simulink model "bh_4dof_LAGR_manipulator"  (R2016a)
settings: Solver=ode15s  StartTime=0.0  StopTime=30  FixedStep=0.001  RelTol=1e-5
values from neighbouring files (symbols this model uses):
  b1_damp = 0.005    [bh_params_single_link_control_explore.m]
  b4_damp = 0.005    [bh_params_single_link_control_explore.m]
  g = 9.80665    [bh_params_single_link_control_explore.m]
  Hz = 0.20    (= 0.2)    [bh_params_single_link_control_explore.m]
  L1x = 1.5    [bh_params_single_link_control_explore.m]
  L1y = 0.050    (= 0.05)    [bh_params_single_link_control_explore.m]
  L1z = 0.005    [bh_params_single_link_control_explore.m]
  mass1 = density * L1x*L1y*L1z    (= 0.375)    [bh_params_single_link_control_explore.m]
  mass4 = density * Hz*pi*(Rturn^2)    (= 1.57079632679)    [bh_params_single_link_control_explore.m]
  Rturn = 0.05    [bh_params_single_link_control_explore.m]
  theta1_0 = 0    [bh_params_single_link_control_explore.m]
  theta1_dot_0 = 0    [bh_params_single_link_control_explore.m]
  theta4_0 = 0    [bh_params_single_link_control_explore.m]
  theta4_dot_0 = 0    [bh_params_single_link_control_explore.m]
undefined symbols (not defined in the file or in its folder): b2_damp, b3_damp, L2x, L2y, L2z, L3x, L3y, L3z, mass2, mass3, theta2_0, theta2_dot_0, theta3_0, theta3_dot_0, X, Y, Z
libraries: sm_lib x26, nesl_utility x17
(part 1 of 2)
settings Model: Creator=bhorton  LastModifiedBy=bhorton
settings SolverCC: ZeroCrossAlgorithm=Adaptive
settings GRTTargetCC: GeneratePreprocessorConditionals=Use local settings
settings SimscapeCC: SimscapeLogType=all  SimscapeLogDataHistory=10000  SelectedTab=Simscape Multibody

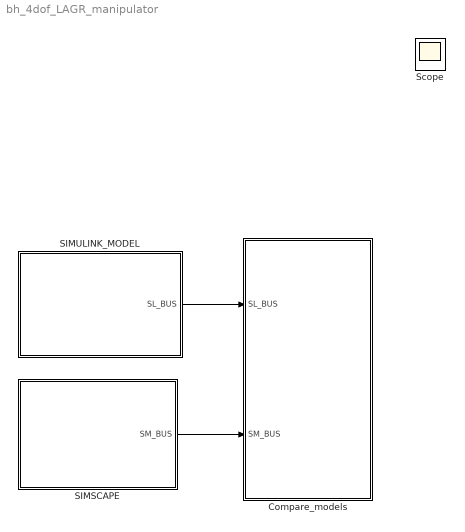
== system bh_4dof_LAGR_manipulator ==
  Compare_models : Subsystem
  SIMSCAPE : Subsystem
  SIMULINK_MODEL : Subsystem
  Scope : Scope
  wires:
  SIMULINK_MODEL/1(SL_BUS) -> Compare_models/1(SL_BUS)
  SIMSCAPE/1(SM_BUS) -> Compare_models/2(SM_BUS)

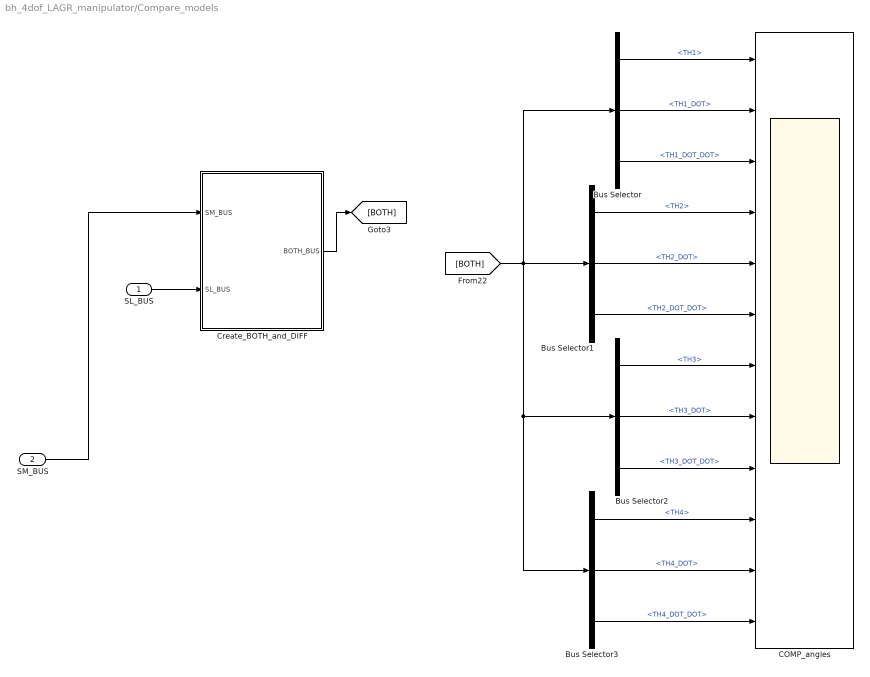
== system bh_4dof_LAGR_manipulator/Compare_models ==
  SL_BUS : Inport
  SM_BUS : Inport  Port=2
  Bus Selector : BusSelector  OutputSignals=TH1,TH1_DOT,TH1_DOT_DOT
  Bus Selector1 : BusSelector  OutputSignals=TH2,TH2_DOT,TH2_DOT_DOT
  Bus Selector2 : BusSelector  OutputSignals=TH3,TH3_DOT,TH3_DOT_DOT
  Bus Selector3 : BusSelector  OutputSignals=TH4,TH4_DOT,TH4_DOT_DOT
  COMP_angles : Scope  NumInputPorts=12
  Create_BOTH_and_DIFF : Subsystem
  wires:
  SM_BUS/1 -> Create_BOTH_and_DIFF/1(SM_BUS)
  SL_BUS/1 -> Create_BOTH_and_DIFF/2(SL_BUS)
  Create_BOTH_and_DIFF/1(BOTH_BUS) -> [BOTH]
  Bus Selector/1 -> COMP_angles/1  "<TH1>"
  Bus Selector/2 -> COMP_angles/2  "<TH1_DOT>"
  Bus Selector/3 -> COMP_angles/3  "<TH1_DOT_DOT>"
  Bus Selector1/1 -> COMP_angles/4  "<TH2>"
  Bus Selector1/2 -> COMP_angles/5  "<TH2_DOT>"
  Bus Selector1/3 -> COMP_angles/6  "<TH2_DOT_DOT>"
  Bus Selector2/1 -> COMP_angles/7  "<TH3>"
  Bus Selector2/2 -> COMP_angles/8  "<TH3_DOT>"
  Bus Selector2/3 -> COMP_angles/9  "<TH3_DOT_DOT>"
  [BOTH] -> Bus Selector/1, Bus Selector3/1, Bus Selector2/1, Bus Selector1/1
  Bus Selector3/1 -> COMP_angles/10  "<TH4>"
  Bus Selector3/2 -> COMP_angles/11  "<TH4_DOT>"
  Bus Selector3/3 -> COMP_angles/12  "<TH4_DOT_DOT>"

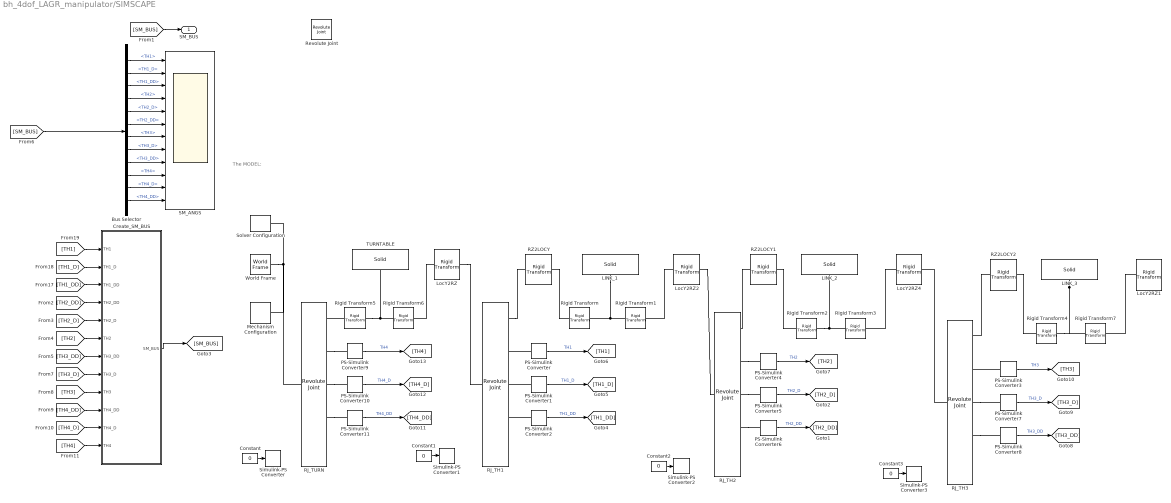
== system bh_4dof_LAGR_manipulator/SIMSCAPE ==
  note: The MODEL:
  Bus Selector : BusSelector  OutputSignals=TH1,TH1_D,TH1_DD,TH2,TH2_D,TH2_DD,TH3,TH3_D,TH3_DD,TH4,TH4_D,TH4_DD
  Constant{,1..3} (4 alike) : Constant  Value=0
  Create_SM_BUS : Subsystem
  LINK_1 : sm_lib/Body Elements/Solid  InertiaType=CalculateFromGeometry  Mass=1  MassUnits=kg  CenterOfMass=[0 0 0]  CenterOfMassUnits=m  MomentsOfInertia=[1 1 1]  MomentsOfInertiaUnits=kg*m^2  ProductsOfInertia=[0 0 0]  ProductsOfInertiaUnits=kg*m^2  DensityBased=on  Density=density  DensityUnits=kg/(m^3)  DoExposeReferenceFrame=on  SerializedFrames=<Frames/>  GraphicType=FromGeometry  MarkerShape=Sphere  MarkerSize=10  GraphicVisPropType=SimpleVisualProperties  GraphicDiffuseColor=[0.2 0.2 1.0]  GraphicSpecularColor=[0.5 0.5 0.5 1.0]  GraphicAmbientColor=[0.15 0.15 0.15 1.0]  GraphicEmissiveColor=[0.0 0.0 0.0 1.0]  GraphicShininess=75  GraphicOpacity=1.0  GeometryShape=Brick  RectangleSize=[1 1]  RectangleSizeUnits=m  BrickDimensions=[L1x, L1y, L1z ]  BrickDimensionUnits=m  CylinderRadius=1  CylinderRadiusUnits=m  CylinderLength=1  CylinderLengthUnits=m  SphereRadius=1  SphereRadiusUnits=m  EllipsoidRadii=[1 1 1]  EllipsoidRadiiUnits=m  ExtrusionCrossSection=[1 1; -1 1; -1 -1; 1 -1]  ExtrusionCrossSectionUnits=m  ExtrusionLength=1  ExtrusionLengthUnits=m  PolygonNumSides=3  PolygonOuterRadius=1  PolygonOuterRadiusUnits=m  ExtGeomFileType=STEP  ExtGeomFileUnits=m  RevolutionCrossSection=[1 1; 1 -1; 2 -1; 2 1]  RevolutionCrossSectionUnits=m  RevolutionExtent=Full  RevolutionAngle=180  RevolutionAngleUnits=deg
  LINK_2 : sm_lib/Body Elements/Solid  InertiaType=CalculateFromGeometry  Mass=1  MassUnits=kg  CenterOfMass=[0 0 0]  CenterOfMassUnits=m  MomentsOfInertia=[1 1 1]  MomentsOfInertiaUnits=kg*m^2  ProductsOfInertia=[0 0 0]  ProductsOfInertiaUnits=kg*m^2  DensityBased=on  Density=density  DensityUnits=kg/(m^3)  DoExposeReferenceFrame=on  SerializedFrames=<Frames/>  GraphicType=FromGeometry  MarkerShape=Sphere  MarkerSize=10  GraphicVisPropType=SimpleVisualProperties  GraphicDiffuseColor=[0.8 0.8 1.0]  GraphicSpecularColor=[0.5 0.5 0.5 1.0]  GraphicAmbientColor=[0.15 0.15 0.15 1.0]  GraphicEmissiveColor=[0.0 0.0 0.0 1.0]  GraphicShininess=75  GraphicOpacity=1.0  GeometryShape=Brick  RectangleSize=[1 1]  RectangleSizeUnits=m  BrickDimensions=[L2x, L2y, L2z ]  BrickDimensionUnits=m  CylinderRadius=1  CylinderRadiusUnits=m  CylinderLength=1  CylinderLengthUnits=m  SphereRadius=1  SphereRadiusUnits=m  EllipsoidRadii=[1 1 1]  EllipsoidRadiiUnits=m  ExtrusionCrossSection=[1 1; -1 1; -1 -1; 1 -1]  ExtrusionCrossSectionUnits=m  ExtrusionLength=1  ExtrusionLengthUnits=m  PolygonNumSides=3  PolygonOuterRadius=1  PolygonOuterRadiusUnits=m  ExtGeomFileType=STEP  ExtGeomFileUnits=m  RevolutionCrossSection=[1 1; 1 -1; 2 -1; 2 1]  RevolutionCrossSectionUnits=m  RevolutionExtent=Full  RevolutionAngle=180  RevolutionAngleUnits=deg
  LINK_3 : sm_lib/Body Elements/Solid  InertiaType=CalculateFromGeometry  Mass=1  MassUnits=kg  CenterOfMass=[0 0 0]  CenterOfMassUnits=m  MomentsOfInertia=[1 1 1]  MomentsOfInertiaUnits=kg*m^2  ProductsOfInertia=[0 0 0]  ProductsOfInertiaUnits=kg*m^2  DensityBased=on  Density=density  DensityUnits=kg/(m^3)  DoExposeReferenceFrame=on  SerializedFrames=<Frames/>  GraphicType=FromGeometry  MarkerShape=Sphere  MarkerSize=10  GraphicVisPropType=SimpleVisualProperties  GraphicDiffuseColor=[1.0 0.8 0.4]  GraphicSpecularColor=[0.5 0.5 0.5 1.0]  GraphicAmbientColor=[0.15 0.15 0.15 1.0]  GraphicEmissiveColor=[0.0 0.0 0.0 1.0]  GraphicShininess=75  GraphicOpacity=1.0  GeometryShape=Brick  RectangleSize=[1 1]  RectangleSizeUnits=m  BrickDimensions=[L3x, L3y, L3z ]  BrickDimensionUnits=m  CylinderRadius=1  CylinderRadiusUnits=m  CylinderLength=1  CylinderLengthUnits=m  SphereRadius=1  SphereRadiusUnits=m  EllipsoidRadii=[1 1 1]  EllipsoidRadiiUnits=m  ExtrusionCrossSection=[1 1; -1 1; -1 -1; 1 -1]  ExtrusionCrossSectionUnits=m  ExtrusionLength=1  ExtrusionLengthUnits=m  PolygonNumSides=3  PolygonOuterRadius=1  PolygonOuterRadiusUnits=m  ExtGeomFileType=STEP  ExtGeomFileUnits=m  RevolutionCrossSection=[1 1; 1 -1; 2 -1; 2 1]  RevolutionCrossSectionUnits=m  RevolutionExtent=Full  RevolutionAngle=180  RevolutionAngleUnits=deg
  LocY2RZ{,1..2,4} (4 alike) : sm_lib/Frames and Transforms/Rigid Transform  TranslationMethod=None  TranslationLengthUnit=m  TranslationStandardAxis=+Z  TranslationStandardOffset=Hz/2  TranslationCartesianOffset=[0 0 0]  TranslationROffset=0  TranslationROffsetUnits=m  TranslationZOffset=0  TranslationZOffsetUnits=m  TranslationThetaOffset=0  TranslationThetaOffsetUnits=deg  RotationMethod=AlignedAxes  RotationAngleUnits=deg  RotationStandardAxis=+Z  RotationAngle=0.0  RotationArbitraryAxis=[0 0 1]  FollAlignAxisA=+X  BaseAlignAxisA=+Y  FollAlignAxisB=+Y  BaseAlignAxisB=+Z  RotationSequenceAxes=FollowerAxes  RotationSequence=XYX  RotationSequenceAngles=[0 0 0]  RotationSequenceAnglesUnits=deg  RotationMatrix=[1 0 0; 0 1 0; 0 0 1]
  Mechanism Configuration : sm_lib/Utilities/Mechanism Configuration  UniformGravity=Constant  GravityVector=[0 0 -9.80665 ]  GravityUnits=m/s^2  LinearizationDelta=1e-4
  PS-Simulink Converter{,3..4,9} (4 alike) : nesl_utility/PS-Simulink Converter  PhysicalDomain=network_engine_domain  SubClassName=ps_output  LeftPortType=input  RightPortType=output  PseudoPeriodic=off  Frequencies=[]  Unit=rad  AffineConversion=off
  PS-Simulink Converter{1,5,7,10} (4 alike) : nesl_utility/PS-Simulink Converter  PhysicalDomain=network_engine_domain  SubClassName=ps_output  LeftPortType=input  RightPortType=output  PseudoPeriodic=off  Frequencies=[]  Unit=rad/s  AffineConversion=off
  PS-Simulink Converter{2,6,8,11} (4 alike) : nesl_utility/PS-Simulink Converter  PhysicalDomain=network_engine_domain  SubClassName=ps_output  LeftPortType=input  RightPortType=output  PseudoPeriodic=off  Frequencies=[]  Unit=rad/s^2  AffineConversion=off
  RJ_TH1 : sm_lib/Joints/Revolute Joint  SenseConstraintForce=on  SenseConstraintForceX=off  SenseConstraintForceY=off  SenseConstraintForceZ=off  SenseConstraintTorque=off  SenseConstraintTorqueX=off  SenseConstraintTorqueY=off  SenseConstraintTorqueZ=off  SenseTotalForce=off  SenseTotalForceX=off  SenseTotalForceY=off  SenseTotalForceZ=off  SenseTotalTorque=off  SenseTotalTorqueX=off  SenseTotalTorqueY=off  SenseTotalTorqueZ=off  CompositeWrenchDir=BaseOnFollower  CompositeWrenchFrame=BaseFrame  EquilibriumPosition=0  EquilibriumPositionUnits=deg  SpringStiffness=0  SpringStiffnessUnits=N*m/deg  DampingCoefficient=b1_damp  DampingCoefficientUnits=N*m/(rad/s)  TorqueActuationMode=NoTorque  MotionActuationMode=ComputedMotion  SensePosition=on  SenseVelocity=on  SenseAcceleration=on  SenseTorqueForce=off  PositionTargetSpecify=on  PositionTargetPriority=Low  PositionTargetValue=theta1_0  PositionTargetValueUnits=rad  VelocityTargetSpecify=on  VelocityTargetPriority=High  VelocityTargetValue=theta1_dot_0  VelocityTargetValueUnits=rad/s
      settings: AttributesFormatString=|
      | %<DampingCoefficient>
      | %<PositionTargetValue>
      | %<VelocityTargetValue>
  RJ_TH2 : sm_lib/Joints/Revolute Joint  SenseConstraintForce=on  SenseConstraintForceX=off  SenseConstraintForceY=off  SenseConstraintForceZ=off  SenseConstraintTorque=off  SenseConstraintTorqueX=off  SenseConstraintTorqueY=off  SenseConstraintTorqueZ=off  SenseTotalForce=off  SenseTotalForceX=off  SenseTotalForceY=off  SenseTotalForceZ=off  SenseTotalTorque=off  SenseTotalTorqueX=off  SenseTotalTorqueY=off  SenseTotalTorqueZ=off  CompositeWrenchDir=BaseOnFollower  CompositeWrenchFrame=BaseFrame  EquilibriumPosition=0  EquilibriumPositionUnits=deg  SpringStiffness=0  SpringStiffnessUnits=N*m/deg  DampingCoefficient=b2_damp  DampingCoefficientUnits=N*m/(rad/s)  TorqueActuationMode=NoTorque  MotionActuationMode=ComputedMotion  SensePosition=on  SenseVelocity=on  SenseAcceleration=on  SenseTorqueForce=off  PositionTargetSpecify=on  PositionTargetPriority=Low  PositionTargetValue=theta2_0  PositionTargetValueUnits=rad  VelocityTargetSpecify=on  VelocityTargetPriority=High  VelocityTargetValue=theta2_dot_0  VelocityTargetValueUnits=rad/s
      settings: AttributesFormatString=|
      | %<DampingCoefficient>
      | %<PositionTargetValue>
      | %<VelocityTargetValue>
  RJ_TH3 : sm_lib/Joints/Revolute Joint  SenseConstraintForce=on  SenseConstraintForceX=off  SenseConstraintForceY=off  SenseConstraintForceZ=off  SenseConstraintTorque=off  SenseConstraintTorqueX=off  SenseConstraintTorqueY=off  SenseConstraintTorqueZ=off  SenseTotalForce=off  SenseTotalForceX=off  SenseTotalForceY=off  SenseTotalForceZ=off  SenseTotalTorque=off  SenseTotalTorqueX=off  SenseTotalTorqueY=off  SenseTotalTorqueZ=off  CompositeWrenchDir=BaseOnFollower  CompositeWrenchFrame=BaseFrame  EquilibriumPosition=0  EquilibriumPositionUnits=deg  SpringStiffness=0  SpringStiffnessUnits=N*m/deg  DampingCoefficient=b3_damp  DampingCoefficientUnits=N*m/(rad/s)  TorqueActuationMode=NoTorque  MotionActuationMode=ComputedMotion  SensePosition=on  SenseVelocity=on  SenseAcceleration=on  SenseTorqueForce=off  PositionTargetSpecify=on  PositionTargetPriority=Low  PositionTargetValue=theta3_0  PositionTargetValueUnits=rad  VelocityTargetSpecify=on  VelocityTargetPriority=High  VelocityTargetValue=theta3_dot_0  VelocityTargetValueUnits=rad/s
      settings: AttributesFormatString=|
      | %<DampingCoefficient>
      | %<PositionTargetValue>
      | %<VelocityTargetValue>
  RJ_TURN : sm_lib/Joints/Revolute Joint  SenseConstraintForce=on  SenseConstraintForceX=off  SenseConstraintForceY=off  SenseConstraintForceZ=off  SenseConstraintTorque=off  SenseConstraintTorqueX=off  SenseConstraintTorqueY=off  SenseConstraintTorqueZ=off  SenseTotalForce=off  SenseTotalForceX=off  SenseTotalForceY=off  SenseTotalForceZ=off  SenseTotalTorque=off  SenseTotalTorqueX=off  SenseTotalTorqueY=off  SenseTotalTorqueZ=off  CompositeWrenchDir=BaseOnFollower  CompositeWrenchFrame=BaseFrame  EquilibriumPosition=0  EquilibriumPositionUnits=deg  SpringStiffness=0  SpringStiffnessUnits=N*m/deg  DampingCoefficient=b4_damp  DampingCoefficientUnits=N*m/(rad/s)  TorqueActuationMode=NoTorque  MotionActuationMode=ComputedMotion  SensePosition=on  SenseVelocity=on  SenseAcceleration=on  SenseTorqueForce=off  PositionTargetSpecify=on  PositionTargetPriority=Low  PositionTargetValue=theta4_0  PositionTargetValueUnits=rad  VelocityTargetSpecify=on  VelocityTargetPriority=High  VelocityTargetValue=theta4_dot_0  VelocityTargetValueUnits=rad/s
      settings: AttributesFormatString=|
      | %<DampingCoefficient>
      | %<PositionTargetValue>
      | %<VelocityTargetValue>
  RZ2LOCY : sm_lib/Frames and Transforms/Rigid Transform  TranslationMethod=None  TranslationLengthUnit=m  TranslationStandardAxis=+Z  TranslationStandardOffset=Hz/2  TranslationCartesianOffset=[0 0 0]  TranslationROffset=0  TranslationROffsetUnits=m  TranslationZOffset=0  TranslationZOffsetUnits=m  TranslationThetaOffset=0  TranslationThetaOffsetUnits=deg  RotationMethod=AlignedAxes  RotationAngleUnits=deg  RotationStandardAxis=+Z  RotationAngle=0.0  RotationArbitraryAxis=[0 0 1]  FollAlignAxisA=+Y  BaseAlignAxisA=+X  FollAlignAxisB=+X  BaseAlignAxisB=+Z  RotationSequenceAxes=FollowerAxes  RotationSequence=XYX  RotationSequenceAngles=[0 0 0]  RotationSequenceAnglesUnits=deg  RotationMatrix=[1 0 0; 0 1 0; 0 0 1]
  RZ2LOCY1 : sm_lib/Frames and Transforms/Rigid Transform  TranslationMethod=None  TranslationLengthUnit=m  TranslationStandardAxis=+Z  TranslationStandardOffset=Hz/2  TranslationCartesianOffset=[0 0 0]  TranslationROffset=0  TranslationROffsetUnits=m  TranslationZOffset=0  TranslationZOffsetUnits=m  TranslationThetaOffset=0  TranslationThetaOffsetUnits=deg  RotationMethod=AlignedAxes  RotationAngleUnits=deg  RotationStandardAxis=+Z  RotationAngle=0.0  RotationArbitraryAxis=[0 0 1]  FollAlignAxisA=+Y  BaseAlignAxisA=+X  FollAlignAxisB=+X  BaseAlignAxisB=+Z  RotationSequenceAxes=FollowerAxes  RotationSequence=XYX  RotationSequenceAngles=[0 0 0]  RotationSequenceAnglesUnits=deg  RotationMatrix=[1 0 0; 0 1 0; 0 0 1]
  RZ2LOCY2 : sm_lib/Frames and Transforms/Rigid Transform  TranslationMethod=None  TranslationLengthUnit=m  TranslationStandardAxis=+Z  TranslationStandardOffset=Hz/2  TranslationCartesianOffset=[0 0 0]  TranslationROffset=0  TranslationROffsetUnits=m  TranslationZOffset=0  TranslationZOffsetUnits=m  TranslationThetaOffset=0  TranslationThetaOffsetUnits=deg  RotationMethod=AlignedAxes  RotationAngleUnits=deg  RotationStandardAxis=+Z  RotationAngle=0.0  RotationArbitraryAxis=[0 0 1]  FollAlignAxisA=+Y  BaseAlignAxisA=+X  FollAlignAxisB=+X  BaseAlignAxisB=+Z  RotationSequenceAxes=FollowerAxes  RotationSequence=XYX  RotationSequenceAngles=[0 0 0]  RotationSequenceAnglesUnits=deg  RotationMatrix=[1 0 0; 0 1 0; 0 0 1]
  Revolute Joint : sm_lib/Joints/Revolute Joint  SenseConstraintForce=off  SenseConstraintForceX=off  SenseConstraintForceY=off  SenseConstraintForceZ=off  SenseConstraintTorque=off  SenseConstraintTorqueX=off  SenseConstraintTorqueY=off  SenseConstraintTorqueZ=off  SenseTotalForce=off  SenseTotalForceX=off  SenseTotalForceY=off  SenseTotalForceZ=off  SenseTotalTorque=off  SenseTotalTorqueX=off  SenseTotalTorqueY=off  SenseTotalTorqueZ=off  CompositeWrenchDir=FollowerOnBase  CompositeWrenchFrame=BaseFrame  EquilibriumPosition=0  EquilibriumPositionUnits=deg  SpringStiffness=0  SpringStiffnessUnits=N*m/deg  DampingCoefficient=0  DampingCoefficientUnits=N*m/(deg/s)  TorqueActuationMode=NoTorque  MotionActuationMode=ComputedMotion  SensePosition=off  SenseVelocity=off  SenseAcceleration=off  SenseTorqueForce=off  PositionTargetSpecify=off  PositionTargetPriority=High  PositionTargetValue=0  PositionTargetValueUnits=deg  VelocityTargetSpecify=off  VelocityTargetPriority=High  VelocityTargetValue=0  VelocityTargetValueUnits=deg/s
  Rigid Transform : sm_lib/Frames and Transforms/Rigid Transform  TranslationMethod=StandardAxis  TranslationLengthUnit=m  TranslationStandardAxis=+Y  TranslationStandardOffset=L1y/2  TranslationCartesianOffset=[0 0 0]  TranslationROffset=0  TranslationROffsetUnits=m  TranslationZOffset=0  TranslationZOffsetUnits=m  TranslationThetaOffset=0  TranslationThetaOffsetUnits=deg  RotationMethod=None  RotationAngleUnits=deg  RotationStandardAxis=+Z  RotationAngle=0.0  RotationArbitraryAxis=[0 0 1]  FollAlignAxisA=+X  BaseAlignAxisA=+Y  FollAlignAxisB=+Y  BaseAlignAxisB=+Z  RotationSequenceAxes=FollowerAxes  RotationSequence=XYX  RotationSequenceAngles=[0 0 0]  RotationSequenceAnglesUnits=deg  RotationMatrix=[1 0 0; 0 1 0; 0 0 1]
  Rigid Transform1 : sm_lib/Frames and Transforms/Rigid Transform  TranslationMethod=StandardAxis  TranslationLengthUnit=m  TranslationStandardAxis=+Y  TranslationStandardOffset=L1y/2  TranslationCartesianOffset=[0 0 0]  TranslationROffset=0  TranslationROffsetUnits=m  TranslationZOffset=0  TranslationZOffsetUnits=m  TranslationThetaOffset=0  TranslationThetaOffsetUnits=deg  RotationMethod=None  RotationAngleUnits=deg  RotationStandardAxis=+Z  RotationAngle=0.0  RotationArbitraryAxis=[0 0 1]  FollAlignAxisA=+X  BaseAlignAxisA=+Y  FollAlignAxisB=+Y  BaseAlignAxisB=+Z  RotationSequenceAxes=FollowerAxes  RotationSequence=XYX  RotationSequenceAngles=[0 0 0]  RotationSequenceAnglesUnits=deg  RotationMatrix=[1 0 0; 0 1 0; 0 0 1]
  Rigid Transform2 : sm_lib/Frames and Transforms/Rigid Transform  TranslationMethod=StandardAxis  TranslationLengthUnit=m  TranslationStandardAxis=+Y  TranslationStandardOffset=L2y/2  TranslationCartesianOffset=[0 0 0]  TranslationROffset=0  TranslationROffsetUnits=m  TranslationZOffset=0  TranslationZOffsetUnits=m  TranslationThetaOffset=0  TranslationThetaOffsetUnits=deg  RotationMethod=None  RotationAngleUnits=deg  RotationStandardAxis=+Z  RotationAngle=0.0  RotationArbitraryAxis=[0 0 1]  FollAlignAxisA=+X  BaseAlignAxisA=+Y  FollAlignAxisB=+Y  BaseAlignAxisB=+Z  RotationSequenceAxes=FollowerAxes  RotationSequence=XYX  RotationSequenceAngles=[0 0 0]  RotationSequenceAnglesUnits=deg  RotationMatrix=[1 0 0; 0 1 0; 0 0 1]
  Rigid Transform3 : sm_lib/Frames and Transforms/Rigid Transform  TranslationMethod=StandardAxis  TranslationLengthUnit=m  TranslationStandardAxis=+Y  TranslationStandardOffset=L2y/2  TranslationCartesianOffset=[0 0 0]  TranslationROffset=0  TranslationROffsetUnits=m  TranslationZOffset=0  TranslationZOffsetUnits=m  TranslationThetaOffset=0  TranslationThetaOffsetUnits=deg  RotationMethod=None  RotationAngleUnits=deg  RotationStandardAxis=+Z  RotationAngle=0.0  RotationArbitraryAxis=[0 0 1]  FollAlignAxisA=+X  BaseAlignAxisA=+Y  FollAlignAxisB=+Y  BaseAlignAxisB=+Z  RotationSequenceAxes=FollowerAxes  RotationSequence=XYX  RotationSequenceAngles=[0 0 0]  RotationSequenceAnglesUnits=deg  RotationMatrix=[1 0 0; 0 1 0; 0 0 1]
  Rigid Transform4 : sm_lib/Frames and Transforms/Rigid Transform  TranslationMethod=StandardAxis  TranslationLengthUnit=m  TranslationStandardAxis=+Y  TranslationStandardOffset=L3y/2  TranslationCartesianOffset=[0 0 0]  TranslationROffset=0  TranslationROffsetUnits=m  TranslationZOffset=0  TranslationZOffsetUnits=m  TranslationThetaOffset=0  TranslationThetaOffsetUnits=deg  RotationMethod=None  RotationAngleUnits=deg  RotationStandardAxis=+Z  RotationAngle=0.0  RotationArbitraryAxis=[0 0 1]  FollAlignAxisA=+X  BaseAlignAxisA=+Y  FollAlignAxisB=+Y  BaseAlignAxisB=+Z  RotationSequenceAxes=FollowerAxes  RotationSequence=XYX  RotationSequenceAngles=[0 0 0]  RotationSequenceAnglesUnits=deg  RotationMatrix=[1 0 0; 0 1 0; 0 0 1]
  Rigid Transform5 : sm_lib/Frames and Transforms/Rigid Transform  TranslationMethod=StandardAxis  TranslationLengthUnit=m  TranslationStandardAxis=-Z  TranslationStandardOffset=Hz/2  TranslationCartesianOffset=[0 0 0]  TranslationROffset=0  TranslationROffsetUnits=m  TranslationZOffset=0  TranslationZOffsetUnits=m  TranslationThetaOffset=0  TranslationThetaOffsetUnits=deg  RotationMethod=None  RotationAngleUnits=deg  RotationStandardAxis=+Z  RotationAngle=0.0  RotationArbitraryAxis=[0 0 1]  FollAlignAxisA=+X  BaseAlignAxisA=+Y  FollAlignAxisB=+Y  BaseAlignAxisB=+Z  RotationSequenceAxes=FollowerAxes  RotationSequence=XYX  RotationSequenceAngles=[0 0 0]  RotationSequenceAnglesUnits=deg  RotationMatrix=[1 0 0; 0 1 0; 0 0 1]
  Rigid Transform6 : sm_lib/Frames and Transforms/Rigid Transform  TranslationMethod=StandardAxis  TranslationLengthUnit=m  TranslationStandardAxis=+Z  TranslationStandardOffset=Hz/2  TranslationCartesianOffset=[0 0 0]  TranslationROffset=0  TranslationROffsetUnits=m  TranslationZOffset=0  TranslationZOffsetUnits=m  TranslationThetaOffset=0  TranslationThetaOffsetUnits=deg  RotationMethod=None  RotationAngleUnits=deg  RotationStandardAxis=+Z  RotationAngle=0.0  RotationArbitraryAxis=[0 0 1]  FollAlignAxisA=+X  BaseAlignAxisA=+Y  FollAlignAxisB=+Y  BaseAlignAxisB=+Z  RotationSequenceAxes=FollowerAxes  RotationSequence=XYX  RotationSequenceAngles=[0 0 0]  RotationSequenceAnglesUnits=deg  RotationMatrix=[1 0 0; 0 1 0; 0 0 1]
  Rigid Transform7 : sm_lib/Frames and Transforms/Rigid Transform  TranslationMethod=StandardAxis  TranslationLengthUnit=m  TranslationStandardAxis=+Y  TranslationStandardOffset=L3y/2  TranslationCartesianOffset=[0 0 0]  TranslationROffset=0  TranslationROffsetUnits=m  TranslationZOffset=0  TranslationZOffsetUnits=m  TranslationThetaOffset=0  TranslationThetaOffsetUnits=deg  RotationMethod=None  RotationAngleUnits=deg  RotationStandardAxis=+Z  RotationAngle=0.0  RotationArbitraryAxis=[0 0 1]  FollAlignAxisA=+X  BaseAlignAxisA=+Y  FollAlignAxisB=+Y  BaseAlignAxisB=+Z  RotationSequenceAxes=FollowerAxes  RotationSequence=XYX  RotationSequenceAngles=[0 0 0]  RotationSequenceAnglesUnits=deg  RotationMatrix=[1 0 0; 0 1 0; 0 0 1]
  SM_ANGS : Scope  NumInputPorts=12
  Simulink-PS Converter{,1..3} (4 alike) : nesl_utility/Simulink-PS Converter  PhysicalDomain=network_engine_domain  SubClassName=ps_input  LeftPortType=input  RightPortType=output  PseudoPeriodic=off  Frequencies=[]  NoiseDistribution=none  NoiseParameters=[]  Unit=N*m  AffineConversion=off  InputFiltering=off  SimscapeFilterOrder=1  InputFilterTimeConstant=0.001  UdotUserProvided=1
  Solver Configuration : nesl_utility/Solver Configuration  PhysicalDomain=network_engine_domain  SubClassName=solver  LeftPortType=input  RightPortType=generic  Accelerate=off  Tones=[]  Harmonics=[]  SimulateNoise=off  Profile=off  UseLocalSampling=off  EnableSwitchedLinearOptims=on  FrequencyDomain=off  UseCCode=off  RelTol=0.001  AbsTol=1e-06  MinStep=1e-09  ToWorkspace=off  RevertToSquareIcSolve=off  NumHomotopyIterations=100  PhasorMode=off  PhasorModeNumHarmonics=1  OverrideAbsTol=off  DoDC=off  ResidualTolerance=1e-09  UseLocalSolver=off  LocalSolverChoice=NE_TRAPEZOIDAL_ADVANCER  LocalSolverSampleTime=0.01  DoFixedCost=off  MaxNonlinIter=3  MaxModeIter=2  LinearAlgebra=Sparse  DelaysMemoryBudget=1024  AutomaticFiltering=off  FilteringTimeConstant=0.001
  TURNTABLE : sm_lib/Body Elements/Solid  InertiaType=CalculateFromGeometry  Mass=1  MassUnits=kg  CenterOfMass=[0 0 0]  CenterOfMassUnits=m  MomentsOfInertia=[1 1 1]  MomentsOfInertiaUnits=kg*m^2  ProductsOfInertia=[0 0 0]  ProductsOfInertiaUnits=kg*m^2  DensityBased=on  Density=1000  DensityUnits=kg/(m^3)  DoExposeReferenceFrame=on  SerializedFrames=<Frames/>  GraphicType=FromGeometry  MarkerShape=Sphere  MarkerSize=10  GraphicVisPropType=SimpleVisualProperties  GraphicDiffuseColor=[1.0 1.0 0.2]  GraphicSpecularColor=[0.5 0.5 0.5 1.0]  GraphicAmbientColor=[0.15 0.15 0.15 1.0]  GraphicEmissiveColor=[0.0 0.0 0.0 1.0]  GraphicShininess=75  GraphicOpacity=1.0  GeometryShape=Cylinder  RectangleSize=[1 1]  RectangleSizeUnits=m  BrickDimensions=[1 1 1]  BrickDimensionUnits=m  CylinderRadius=Rturn  CylinderRadiusUnits=m  CylinderLength=Hz  CylinderLengthUnits=m  SphereRadius=1  SphereRadiusUnits=m  EllipsoidRadii=[1 1 1]  EllipsoidRadiiUnits=m  ExtrusionCrossSection=[1 1; -1 1; -1 -1; 1 -1]  ExtrusionCrossSectionUnits=m  ExtrusionLength=1  ExtrusionLengthUnits=m  PolygonNumSides=3  PolygonOuterRadius=1  PolygonOuterRadiusUnits=m  ExtGeomFileType=STEP  ExtGeomFileUnits=m  RevolutionCrossSection=[1 1; 1 -1; 2 -1; 2 1]  RevolutionCrossSectionUnits=m  RevolutionExtent=Full  RevolutionAngle=180  RevolutionAngleUnits=deg
  World Frame : sm_lib/Frames and Transforms/World Frame
  SM_BUS : Outport
  wires:
  [SM_BUS] -> SM_BUS/1
  [TH2_D] -> Create_SM_BUS/5(TH2_D)
  [TH1_D] -> Create_SM_BUS/2(TH1_D)
  [TH2_DD] -> Create_SM_BUS/4(TH2_DD)
  [TH2] -> Create_SM_BUS/6(TH2)
  [TH1_DD] -> Create_SM_BUS/3(TH1_DD)
  [TH1] -> Create_SM_BUS/1(TH1)
  Create_SM_BUS/1(SM_BUS) -> [SM_BUS]
  Bus Selector/2 -> SM_ANGS/2  "<TH1_D>"
  Bus Selector/3 -> SM_ANGS/3  "<TH1_DD>"
  Bus Selector/1 -> SM_ANGS/1  "<TH1>"
  Bus Selector/4 -> SM_ANGS/4  "<TH2>"
  Bus Selector/5 -> SM_ANGS/5  "<TH2_D>"
  Bus Selector/6 -> SM_ANGS/6  "<TH2_DD>"
  Bus Selector/7 -> SM_ANGS/7  "<TH3>"
  Bus Selector/8 -> SM_ANGS/8  "<TH3_D>"
  Bus Selector/9 -> SM_ANGS/9  "<TH3_DD>"
  [TH3_DD] -> Create_SM_BUS/7(TH3_DD)
  [TH3_D] -> Create_SM_BUS/8(TH3_D)
  [TH3] -> Create_SM_BUS/9(TH3)
  PS-Simulink Converter/1 -> [TH1]  "TH1"
  PS-Simulink Converter2/1 -> [TH1_DD]  "TH1_DD"
  PS-Simulink Converter1/1 -> [TH1_D]  "TH1_D"
  PS-Simulink Converter4/1 -> [TH2]  "TH2"
  PS-Simulink Converter6/1 -> [TH2_DD]  "TH2_DD"
  PS-Simulink Converter5/1 -> [TH2_D]  "TH2_D"
  PS-Simulink Converter3/1 -> [TH3]  "TH3"
  PS-Simulink Converter8/1 -> [TH3_DD]  "TH3_DD"
  PS-Simulink Converter7/1 -> [TH3_D]  "TH3_D"
  PS-Simulink Converter9/1 -> [TH4]  "TH4"
  PS-Simulink Converter11/1 -> [TH4_DD]  "TH4_DD"
  PS-Simulink Converter10/1 -> [TH4_D]  "TH4_D"
  [TH4_DD] -> Create_SM_BUS/10(TH4_DD)
  [TH4_D] -> Create_SM_BUS/11(TH4_D)
  [TH4] -> Create_SM_BUS/12(TH4)
  Bus Selector/12 -> SM_ANGS/12  "<TH4_DD>"
  Bus Selector/11 -> SM_ANGS/11  "<TH4_D>"
  Bus Selector/10 -> SM_ANGS/10  "<TH4>"
  [SM_BUS] -> Bus Selector/1
  Constant/1 -> Simulink-PS Converter/1
  Constant1/1 -> Simulink-PS Converter1/1
  Constant2/1 -> Simulink-PS Converter2/1
  Constant3/1 -> Simulink-PS Converter3/1
  connections:
  World Frame/RConn1 -- RJ_TURN/LConn1 -- Mechanism Configuration/RConn1 -- Solver Configuration/RConn1
  PS-Simulink Converter1/LConn1 -- RJ_TH1/RConn3
  PS-Simulink Converter2/LConn1 -- RJ_TH1/RConn4
  PS-Simulink Converter/LConn1 -- RJ_TH1/RConn2
  Rigid Transform5/LConn1 -- RJ_TURN/RConn1
  Rigid Transform5/RConn1 -- Rigid Transform6/LConn1 -- TURNTABLE/RConn1
  LocY2RZ/LConn1 -- Rigid Transform6/RConn1
  LocY2RZ/RConn1 -- RJ_TH1/LConn1
  Rigid Transform1/LConn1 -- LINK_1/RConn1 -- Rigid Transform/RConn1
  LocY2RZ2/LConn1 -- Rigid Transform1/RConn1
  LocY2RZ2/RConn1 -- RJ_TH2/LConn1
  RZ2LOCY1/LConn1 -- RJ_TH2/RConn1
  Rigid Transform2/RConn1 -- Rigid Transform3/LConn1 -- LINK_2/RConn1
  LocY2RZ4/LConn1 -- Rigid Transform3/RConn1
  RJ_TH1/RConn1 -- RZ2LOCY/LConn1
  RZ2LOCY/RConn1 -- Rigid Transform/LConn1
  RZ2LOCY1/RConn1 -- Rigid Transform2/LConn1
  RJ_TH3/LConn1 -- LocY2RZ4/RConn1
  LINK_3/RConn1 -- Rigid Transform7/LConn1 -- Rigid Transform4/RConn1
  LocY2RZ1/LConn1 -- Rigid Transform7/RConn1
  RZ2LOCY2/RConn1 -- Rigid Transform4/LConn1
  RZ2LOCY2/LConn1 -- RJ_TH3/RConn1
  RJ_TH2/RConn3 -- PS-Simulink Converter5/LConn1
  RJ_TH2/RConn2 -- PS-Simulink Converter4/LConn1
  RJ_TH2/RConn4 -- PS-Simulink Converter6/LConn1
  PS-Simulink Converter3/LConn1 -- RJ_TH3/RConn2
  RJ_TH3/RConn3 -- PS-Simulink Converter7/LConn1
  RJ_TH3/RConn4 -- PS-Simulink Converter8/LConn1
  RJ_TURN/RConn4 -- PS-Simulink Converter11/LConn1
  RJ_TURN/RConn3 -- PS-Simulink Converter10/LConn1
  RJ_TURN/RConn2 -- PS-Simulink Converter9/LConn1

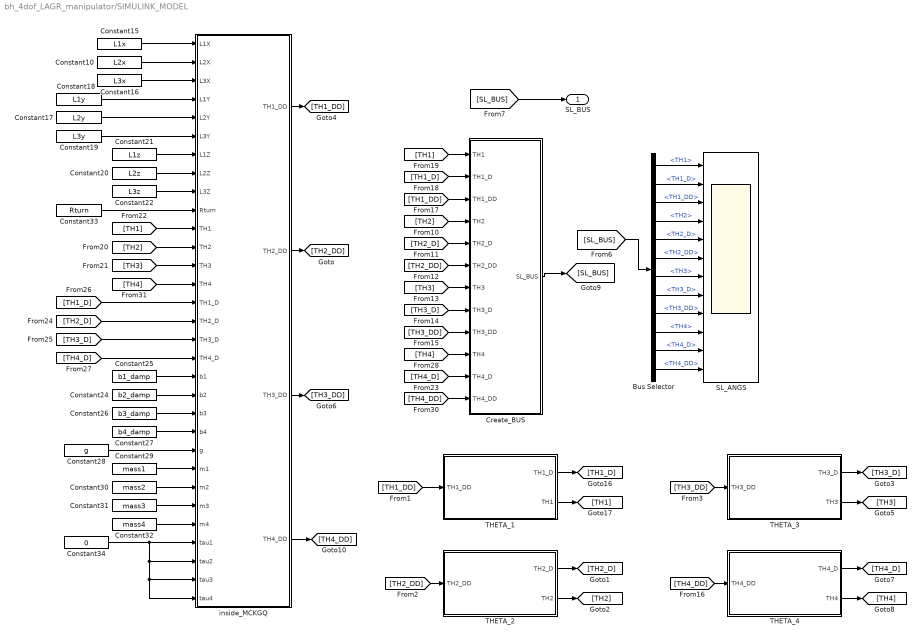
== system bh_4dof_LAGR_manipulator/SIMULINK_MODEL ==
  Bus Selector : BusSelector  OutputSignals=TH1,TH1_D,TH1_DD,TH2,TH2_D,TH2_DD,TH3,TH3_D,TH3_DD,TH4,TH4_D,TH4_DD
  Constant10 : Constant  Value=L2x
  Constant15 : Constant  Value=L1x
  Constant16 : Constant  Value=L3x
  Constant17 : Constant  Value=L2y
  Constant18 : Constant  Value=L1y
  Constant19 : Constant  Value=L3y
  Constant20 : Constant  Value=L2z
  Constant21 : Constant  Value=L1z
  Constant22 : Constant  Value=L3z
  Constant24 : Constant  Value=b2_damp
  Constant25 : Constant  Value=b1_damp
  Constant26 : Constant  Value=b3_damp
  Constant27 : Constant  Value=b4_damp
  Constant28 : Constant  Value=g
  Constant29 : Constant  Value=mass1
  Constant30 : Constant  Value=mass2
  Constant31 : Constant  Value=mass3
  Constant32 : Constant  Value=mass4
  Constant33 : Constant  Value=Rturn
  Constant34 : Constant  Value=0
  Create_BUS : Subsystem
  SL_ANGS : Scope  NumInputPorts=12
  THETA_1 : Subsystem
  THETA_2 : Subsystem
  THETA_3 : Subsystem
  THETA_4 : Subsystem
  inside_MCKGQ : Subsystem
  SL_BUS : Outport
  wires:
  [SL_BUS] -> Bus Selector/1
  [SL_BUS] -> SL_BUS/1
  Create_BUS/1(SL_BUS) -> [SL_BUS]
  Bus Selector/2 -> SL_ANGS/2  "<TH1_D>"
  Bus Selector/3 -> SL_ANGS/3  "<TH1_DD>"
  Bus Selector/1 -> SL_ANGS/1  "<TH1>"
  Bus Selector/4 -> SL_ANGS/4  "<TH2>"
  Bus Selector/5 -> SL_ANGS/5  "<TH2_D>"
  Bus Selector/6 -> SL_ANGS/6  "<TH2_DD>"
  Bus Selector/7 -> SL_ANGS/7  "<TH3>"
  Bus Selector/8 -> SL_ANGS/8  "<TH3_D>"
  Bus Selector/9 -> SL_ANGS/9  "<TH3_DD>"
  [TH2_DD] -> THETA_2/1(TH2_DD)
  THETA_2/2(TH2) -> [TH2]
  THETA_2/1(TH2_D) -> [TH2_D]
  [TH1_DD] -> THETA_1/1(TH1_DD)
  THETA_1/1(TH1_D) -> [TH1_D]
  THETA_1/2(TH1) -> [TH1]
  inside_MCKGQ/2(TH2_DD) -> [TH2_DD]
  [TH3_DD] -> THETA_3/1(TH3_DD)
  THETA_3/2(TH3) -> [TH3]
  THETA_3/1(TH3_D) -> [TH3_D]
  inside_MCKGQ/1(TH1_DD) -> [TH1_DD]
  inside_MCKGQ/3(TH3_DD) -> [TH3_DD]
  [TH3_DD] -> Create_BUS/9(TH3_DD)
  [TH1] -> Create_BUS/1(TH1)
  [TH1_D] -> Create_BUS/2(TH1_D)
  [TH1_DD] -> Create_BUS/3(TH1_DD)
  [TH2] -> Create_BUS/4(TH2)
  [TH2_D] -> Create_BUS/5(TH2_D)
  [TH2_DD] -> Create_BUS/6(TH2_DD)
  [TH3] -> Create_BUS/7(TH3)
  [TH3_D] -> Create_BUS/8(TH3_D)
  [TH4_DD] -> THETA_4/1(TH4_DD)
  THETA_4/2(TH4) -> [TH4]
  THETA_4/1(TH4_D) -> [TH4_D]
  [TH2] -> inside_MCKGQ/12(TH2)
  [TH3] -> inside_MCKGQ/13(TH3)
  [TH1] -> inside_MCKGQ/11(TH1)
  Constant10/1 -> inside_MCKGQ/2(L2X)
  Constant16/1 -> inside_MCKGQ/3(L3X)
  Constant15/1 -> inside_MCKGQ/1(L1X)
  Constant19/1 -> inside_MCKGQ/6(L3Y)
  Constant17/1 -> inside_MCKGQ/5(L2Y)
  Constant18/1 -> inside_MCKGQ/4(L1Y)
  Constant22/1 -> inside_MCKGQ/9(L3Z)
  Constant20/1 -> inside_MCKGQ/8(L2Z)
  Constant21/1 -> inside_MCKGQ/7(L1Z)
  [TH1_D] -> inside_MCKGQ/15(TH1_D)
  [TH2_D] -> inside_MCKGQ/16(TH2_D)
  [TH3_D] -> inside_MCKGQ/17(TH3_D)
  [TH4_D] -> inside_MCKGQ/18(TH4_D)
  Constant25/1 -> inside_MCKGQ/19(b1)
  Constant24/1 -> inside_MCKGQ/20(b2)
  Constant26/1 -> inside_MCKGQ/21(b3)
  Constant27/1 -> inside_MCKGQ/22(b4)
  Constant28/1 -> inside_MCKGQ/23(g)
  Constant29/1 -> inside_MCKGQ/24(m1)
  Constant30/1 -> inside_MCKGQ/25(m2)
  Constant31/1 -> inside_MCKGQ/26(m3)
  Constant32/1 -> inside_MCKGQ/27(m4)
  Constant33/1 -> inside_MCKGQ/10(Rturn)
  Constant34/1 -> inside_MCKGQ/28(tau1), inside_MCKGQ/29(tau2), inside_MCKGQ/31(tau4), inside_MCKGQ/30(tau3)
  [TH4_D] -> Create_BUS/11(TH4_D)
  [TH4_DD] -> Create_BUS/12(TH4_DD)
  [TH4] -> Create_BUS/10(TH4)
  [TH4] -> inside_MCKGQ/14(TH4)
  inside_MCKGQ/4(TH4_DD) -> [TH4_DD]
  Bus Selector/10 -> SL_ANGS/10  "<TH4>"
  Bus Selector/11 -> SL_ANGS/11  "<TH4_D>"
  Bus Selector/12 -> SL_ANGS/12  "<TH4_DD>"

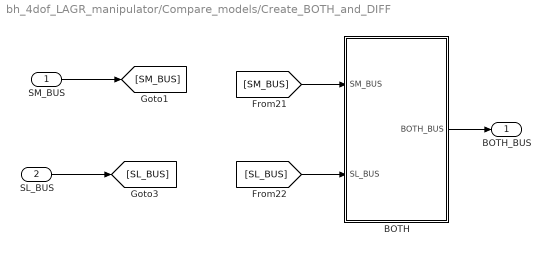
== system bh_4dof_LAGR_manipulator/Compare_models/Create_BOTH_and_DIFF ==
  SM_BUS : Inport
  SL_BUS : Inport  Port=2
  BOTH : Subsystem
  BOTH_BUS : Outport
  wires:
  SL_BUS/1 -> [SL_BUS]
  SM_BUS/1 -> [SM_BUS]
  [SM_BUS] -> BOTH/1(SM_BUS)
  [SL_BUS] -> BOTH/2(SL_BUS)
  BOTH/1(BOTH_BUS) -> BOTH_BUS/1

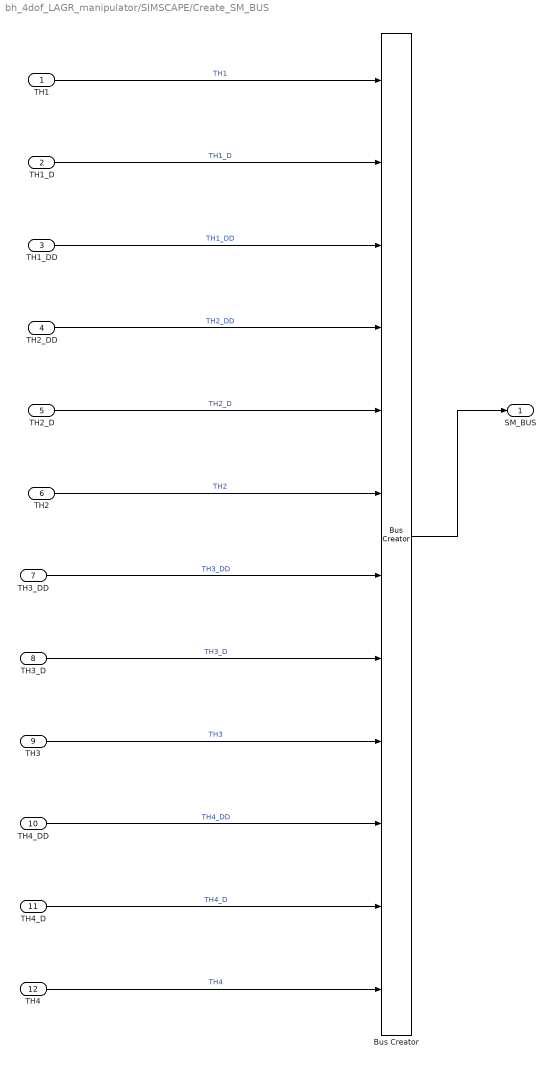
== system bh_4dof_LAGR_manipulator/SIMSCAPE/Create_SM_BUS ==
  TH1 : Inport
  TH1_D : Inport  Port=2
  TH1_DD : Inport  Port=3
  TH2_DD : Inport  Port=4
  TH2_D : Inport  Port=5
  TH2 : Inport  Port=6
  TH3_DD : Inport  Port=7
  TH3_D : Inport  Port=8
  TH3 : Inport  Port=9
  TH4_DD : Inport  Port=10
  TH4_D : Inport  Port=11
  TH4 : Inport  Port=12
  Bus Creator : BusCreator  Inputs=12
  SM_BUS : Outport
  wires:
  TH2_DD/1 -> Bus Creator/4  "TH2_DD"
  TH1_DD/1 -> Bus Creator/3  "TH1_DD"
  TH1_D/1 -> Bus Creator/2  "TH1_D"
  TH2_D/1 -> Bus Creator/5  "TH2_D"
  TH1/1 -> Bus Creator/1  "TH1"
  TH2/1 -> Bus Creator/6  "TH2"
  Bus Creator/1 -> SM_BUS/1
  TH3/1 -> Bus Creator/9  "TH3"
  TH3_D/1 -> Bus Creator/8  "TH3_D"
  TH3_DD/1 -> Bus Creator/7  "TH3_DD"
  TH4/1 -> Bus Creator/12  "TH4"
  TH4_D/1 -> Bus Creator/11  "TH4_D"
  TH4_DD/1 -> Bus Creator/10  "TH4_DD"

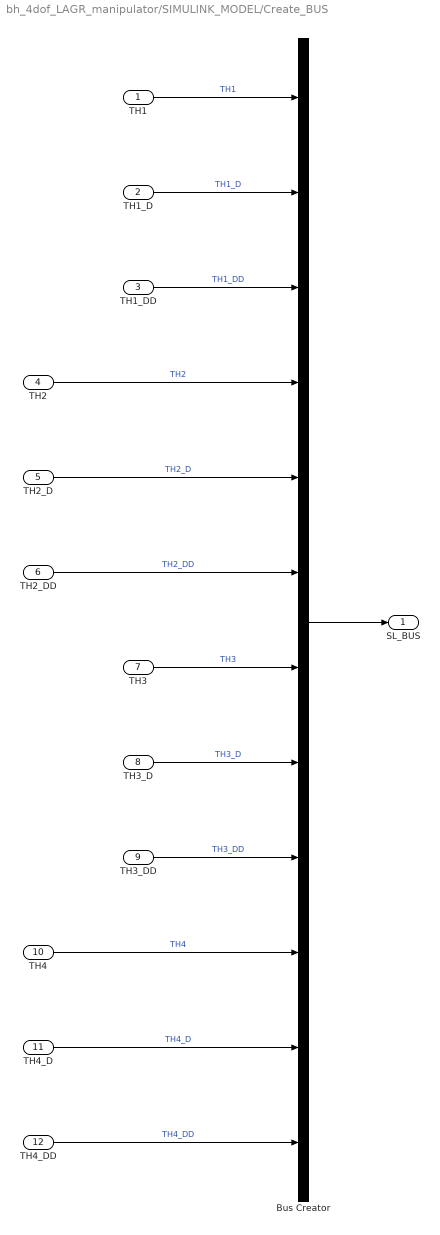
== system bh_4dof_LAGR_manipulator/SIMULINK_MODEL/Create_BUS ==
  TH1 : Inport
  TH1_D : Inport  Port=2
  TH1_DD : Inport  Port=3
  TH2 : Inport  Port=4
  TH2_D : Inport  Port=5
  TH2_DD : Inport  Port=6
  TH3 : Inport  Port=7
  TH3_D : Inport  Port=8
  TH3_DD : Inport  Port=9
  TH4 : Inport  Port=10
  TH4_D : Inport  Port=11
  TH4_DD : Inport  Port=12
  Bus Creator : BusCreator  Inputs=12
  SL_BUS : Outport
  wires:
  TH1_DD/1 -> Bus Creator/3  "TH1_DD"
  TH1_D/1 -> Bus Creator/2  "TH1_D"
  TH1/1 -> Bus Creator/1  "TH1"
  Bus Creator/1 -> SL_BUS/1
  TH2/1 -> Bus Creator/4  "TH2"
  TH2_D/1 -> Bus Creator/5  "TH2_D"
  TH2_DD/1 -> Bus Creator/6  "TH2_DD"
  TH3/1 -> Bus Creator/7  "TH3"
  TH3_DD/1 -> Bus Creator/9  "TH3_DD"
  TH3_D/1 -> Bus Creator/8  "TH3_D"
  TH4_DD/1 -> Bus Creator/12  "TH4_DD"
  TH4_D/1 -> Bus Creator/11  "TH4_D"
  TH4/1 -> Bus Creator/10  "TH4"

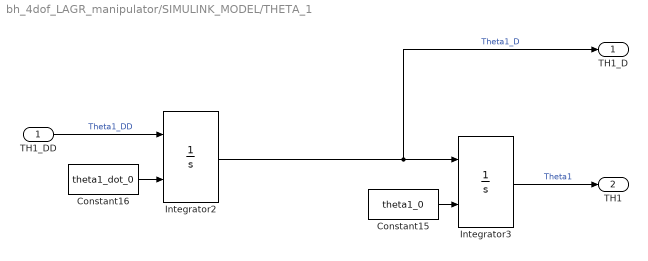
== system bh_4dof_LAGR_manipulator/SIMULINK_MODEL/THETA_1 ==
  TH1_DD : Inport
  Constant15 : Constant  Value=theta1_0
  Constant16 : Constant  Value=theta1_dot_0
  Integrator2 : Integrator  InitialConditionSource=external
  Integrator3 : Integrator  InitialConditionSource=external
  TH1_D : Outport
  TH1 : Outport  Port=2
  wires:
  TH1_DD/1 -> Integrator2/1  "Theta1_DD"
  Constant15/1 -> Integrator3/2
  Constant16/1 -> Integrator2/2
  Integrator3/1 -> TH1/1  "Theta1"
  Integrator2/1 -> TH1_D/1, Integrator3/1  "Theta1_D"

== system bh_4dof_LAGR_manipulator/SIMULINK_MODEL/THETA_2 ==
  TH2_DD : Inport
  Constant15 : Constant  Value=theta2_0
  Constant16 : Constant  Value=theta2_dot_0
  Integrator2 : Integrator  InitialConditionSource=external
  Integrator3 : Integrator  InitialConditionSource=external
  TH2_D : Outport
  TH2 : Outport  Port=2
  wires:
  TH2_DD/1 -> Integrator2/1  "Theta2_DD"
  Integrator2/1 -> TH2_D/1, Integrator3/1  "Theta2_D"
  Constant15/1 -> Integrator3/2
  Constant16/1 -> Integrator2/2
  Integrator3/1 -> TH2/1  "Theta2"

== system bh_4dof_LAGR_manipulator/SIMULINK_MODEL/THETA_3 ==
  TH3_DD : Inport
  Constant15 : Constant  Value=theta3_0
  Constant16 : Constant  Value=theta3_dot_0
  Integrator2 : Integrator  InitialConditionSource=external
  Integrator3 : Integrator  InitialConditionSource=external
  TH3_D : Outport
  TH3 : Outport  Port=2
  wires:
  TH3_DD/1 -> Integrator2/1  "Theta3_DD"
  Integrator2/1 -> TH3_D/1, Integrator3/1  "Theta3_D"
  Constant15/1 -> Integrator3/2
  Constant16/1 -> Integrator2/2
  Integrator3/1 -> TH3/1  "Theta3"

== system bh_4dof_LAGR_manipulator/SIMULINK_MODEL/THETA_4 ==
  TH4_DD : Inport
  Constant15 : Constant  Value=theta4_0
  Constant16 : Constant  Value=theta4_dot_0
  Integrator2 : Integrator  InitialConditionSource=external
  Integrator3 : Integrator  InitialConditionSource=external
  TH4_D : Outport
  TH4 : Outport  Port=2
  wires:
  TH4_DD/1 -> Integrator2/1  "Theta4_DD"
  Integrator2/1 -> TH4_D/1, Integrator3/1  "Theta4_D"
  Constant15/1 -> Integrator3/2
  Constant16/1 -> Integrator2/2
  Integrator3/1 -> TH4/1  "Theta4"

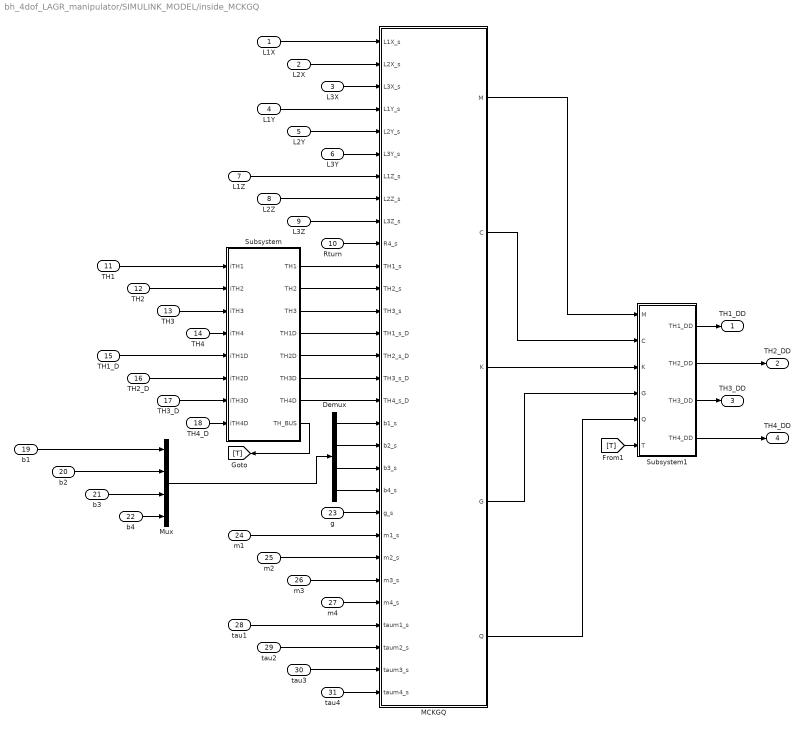
== system bh_4dof_LAGR_manipulator/SIMULINK_MODEL/inside_MCKGQ ==
  L1X : Inport
  L2X : Inport  Port=2
  L3X : Inport  Port=3
  L1Y : Inport  Port=4
  L2Y : Inport  Port=5
  L3Y : Inport  Port=6
  L1Z : Inport  Port=7
  L2Z : Inport  Port=8
  L3Z : Inport  Port=9
  Rturn : Inport  Port=10
  TH1 : Inport  Port=11
  TH2 : Inport  Port=12
  TH3 : Inport  Port=13
  TH4 : Inport  Port=14
  TH1_D : Inport  Port=15
  TH2_D : Inport  Port=16
  TH3_D : Inport  Port=17
  TH4_D : Inport  Port=18
  b1 : Inport  Port=19
  b2 : Inport  Port=20
  b3 : Inport  Port=21
  b4 : Inport  Port=22
  g : Inport  Port=23
  m1 : Inport  Port=24
  m2 : Inport  Port=25
  m3 : Inport  Port=26
  m4 : Inport  Port=27
  tau1 : Inport  Port=28
  tau2 : Inport  Port=29
  tau3 : Inport  Port=30
  tau4 : Inport  Port=31
  Demux : Demux
  MCKGQ : MATLAB Function  TreatAsAtomicUnit=on
  Mux : Mux
  Subsystem : Subsystem
  Subsystem1 : Subsystem
  TH1_DD : Outport
  TH2_DD : Outport  Port=2
  TH3_DD : Outport  Port=3
  TH4_DD : Outport  Port=4
  wires:
  m2/1 -> MCKGQ/24(m2_s)
  m3/1 -> MCKGQ/25(m3_s)
  m4/1 -> MCKGQ/26(m4_s)
  tau1/1 -> MCKGQ/27(taum1_s)
  g/1 -> MCKGQ/22(g_s)
  m1/1 -> MCKGQ/23(m1_s)
  TH1_D/1 -> Subsystem/5(iTH1D)
  b1/1 -> Mux/1
  b2/1 -> Mux/2
  TH3/1 -> Subsystem/3(iTH3)
  b3/1 -> Mux/3
  TH4_D/1 -> Subsystem/8(iTH4D)
  TH2_D/1 -> Subsystem/6(iTH2D)
  TH3_D/1 -> Subsystem/7(iTH3D)
  b4/1 -> Mux/4
  tau2/1 -> MCKGQ/28(taum2_s)
  tau3/1 -> MCKGQ/29(taum3_s)
  tau4/1 -> MCKGQ/30(taum4_s)
  L2X/1 -> MCKGQ/2(L2X_s)
  L3X/1 -> MCKGQ/3(L3X_s)
  L2Y/1 -> MCKGQ/5(L2Y_s)
  L3Y/1 -> MCKGQ/6(L3Y_s)
  L1Y/1 -> MCKGQ/4(L1Y_s)
  L2Z/1 -> MCKGQ/8(L2Z_s)
  L3Z/1 -> MCKGQ/9(L3Z_s)
  L1Z/1 -> MCKGQ/7(L1Z_s)
  TH1/1 -> Subsystem/1(iTH1)
  Rturn/1 -> MCKGQ/10(R4_s)
  TH2/1 -> Subsystem/2(iTH2)
  L1X/1 -> MCKGQ/1(L1X_s)
  Subsystem/8(TH_BUS) -> [T]
  Subsystem/7(TH4D) -> MCKGQ/17(TH4_s_D)
  Subsystem/6(TH3D) -> MCKGQ/16(TH3_s_D)
  Subsystem/5(TH2D) -> MCKGQ/15(TH2_s_D)
  Subsystem/4(TH1D) -> MCKGQ/14(TH1_s_D)
  Subsystem/3(TH3) -> MCKGQ/13(TH3_s)
  Subsystem/2(TH2) -> MCKGQ/12(TH2_s)
  Subsystem/1(TH1) -> MCKGQ/11(TH1_s)
  TH4/1 -> Subsystem/4(iTH4)
  Demux/1 -> MCKGQ/18(b1_s)
  Demux/2 -> MCKGQ/19(b2_s)
  Demux/3 -> MCKGQ/20(b3_s)
  Demux/4 -> MCKGQ/21(b4_s)
  Mux/1 -> Demux/1
  Subsystem1/1(TH1_DD) -> TH1_DD/1
  Subsystem1/2(TH2_DD) -> TH2_DD/1
  MCKGQ/1(M) -> Subsystem1/1(M)
  MCKGQ/2(C) -> Subsystem1/2(C)
  MCKGQ/3(K) -> Subsystem1/3(K)
  MCKGQ/4(G) -> Subsystem1/4(G)
  MCKGQ/5(Q) -> Subsystem1/5(Q)
  [T] -> Subsystem1/6(T)
  Subsystem1/3(TH3_DD) -> TH3_DD/1
  Subsystem1/4(TH4_DD) -> TH4_DD/1

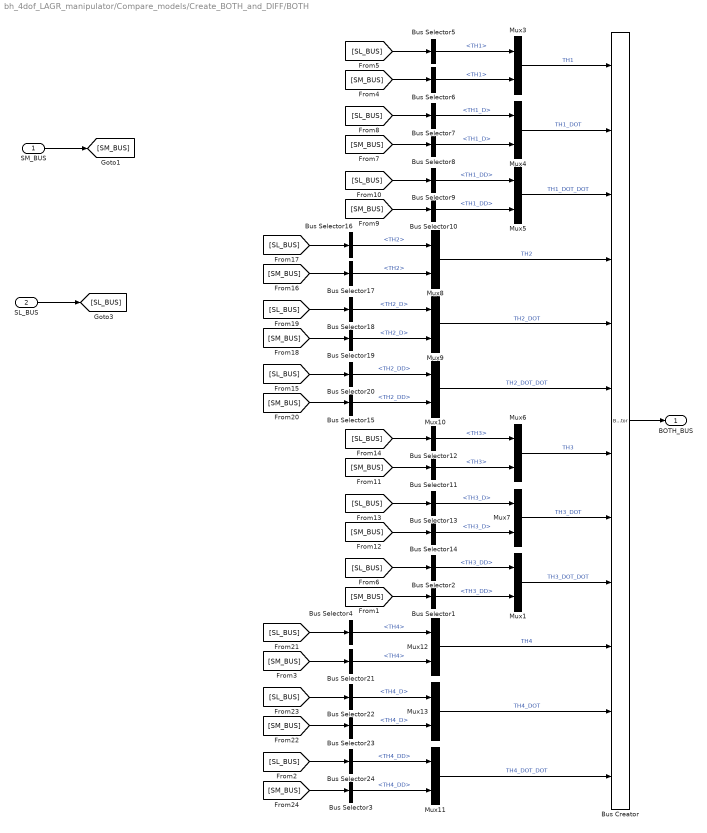
== system bh_4dof_LAGR_manipulator/Compare_models/Create_BOTH_and_DIFF/BOTH ==
  SM_BUS : Inport
  SL_BUS : Inport  Port=2
  Bus Creator : BusCreator  Inputs=12
  Bus Selector1 : BusSelector  OutputSignals=TH3_DD
  Bus Selector10 : BusSelector  OutputSignals=TH1_DD
  Bus Selector11 : BusSelector  OutputSignals=TH3
  Bus Selector12 : BusSelector  OutputSignals=TH3
  Bus Selector13 : BusSelector  OutputSignals=TH3_D
  Bus Selector14 : BusSelector  OutputSignals=TH3_D
  Bus Selector15 : BusSelector  OutputSignals=TH2_DD
  Bus Selector16 : BusSelector  OutputSignals=TH2
  Bus Selector17 : BusSelector  OutputSignals=TH2
  Bus Selector18 : BusSelector  OutputSignals=TH2_D
  Bus Selector19 : BusSelector  OutputSignals=TH2_D
  Bus Selector2 : BusSelector  OutputSignals=TH3_DD
  Bus Selector20 : BusSelector  OutputSignals=TH2_DD
  Bus Selector21 : BusSelector  OutputSignals=TH4
  Bus Selector22 : BusSelector  OutputSignals=TH4_D
  Bus Selector23 : BusSelector  OutputSignals=TH4_D
  Bus Selector24 : BusSelector  OutputSignals=TH4_DD
  Bus Selector3 : BusSelector  OutputSignals=TH4_DD
  Bus Selector4 : BusSelector  OutputSignals=TH4
  Bus Selector5 : BusSelector  OutputSignals=TH1
  Bus Selector6 : BusSelector  OutputSignals=TH1
  Bus Selector7 : BusSelector  OutputSignals=TH1_D
  Bus Selector8 : BusSelector  OutputSignals=TH1_D
  Bus Selector9 : BusSelector  OutputSignals=TH1_DD
  Mux{1,3..13} (12 alike) : Mux  Inputs=2
  BOTH_BUS : Outport
  wires:
  SL_BUS/1 -> [SL_BUS]
  SM_BUS/1 -> [SM_BUS]
  [SL_BUS] -> Bus Selector2/1
  [SM_BUS] -> Bus Selector1/1
  [SM_BUS] -> Bus Selector6/1
  [SL_BUS] -> Bus Selector5/1
  [SL_BUS] -> Bus Selector7/1
  [SM_BUS] -> Bus Selector8/1
  [SL_BUS] -> Bus Selector9/1
  [SM_BUS] -> Bus Selector10/1
  Bus Selector1/1 -> Mux1/2  "<TH3_DD>"
  Bus Selector2/1 -> Mux1/1  "<TH3_DD>"
  Bus Selector5/1 -> Mux3/1  "<TH1>"
  Bus Selector6/1 -> Mux3/2  "<TH1>"
  Bus Selector7/1 -> Mux4/1  "<TH1_D>"
  Bus Selector8/1 -> Mux4/2  "<TH1_D>"
  Bus Selector9/1 -> Mux5/1  "<TH1_DD>"
  Bus Selector10/1 -> Mux5/2  "<TH1_DD>"
  Mux1/1 -> Bus Creator/9  "TH3_DOT_DOT"
  Mux3/1 -> Bus Creator/1  "TH1"
  Mux4/1 -> Bus Creator/2  "TH1_DOT"
  Bus Creator/1 -> BOTH_BUS/1
  Mux5/1 -> Bus Creator/3  "TH1_DOT_DOT"
  [SL_BUS] -> Bus Selector12/1
  [SM_BUS] -> Bus Selector11/1
  [SL_BUS] -> Bus Selector13/1
  Bus Selector11/1 -> Mux6/2  "<TH3>"
  Bus Selector12/1 -> Mux6/1  "<TH3>"
  Bus Selector13/1 -> Mux7/1  "<TH3_D>"
  Mux6/1 -> Bus Creator/7  "TH3"
  Mux7/1 -> Bus Creator/8  "TH3_DOT"
  [SM_BUS] -> Bus Selector14/1
  Bus Selector14/1 -> Mux7/2  "<TH3_D>"
  [SM_BUS] -> Bus Selector17/1
  [SL_BUS] -> Bus Selector16/1
  [SL_BUS] -> Bus Selector18/1
  [SM_BUS] -> Bus Selector19/1
  [SL_BUS] -> Bus Selector20/1
  [SM_BUS] -> Bus Selector15/1
  Bus Selector16/1 -> Mux8/1  "<TH2>"
  Bus Selector17/1 -> Mux8/2  "<TH2>"
  Bus Selector18/1 -> Mux9/1  "<TH2_D>"
  Bus Selector19/1 -> Mux9/2  "<TH2_D>"
  Bus Selector20/1 -> Mux10/1  "<TH2_DD>"
  Bus Selector15/1 -> Mux10/2  "<TH2_DD>"
  Mux8/1 -> Bus Creator/4  "TH2"
  Mux9/1 -> Bus Creator/5  "TH2_DOT"
  Mux10/1 -> Bus Creator/6  "TH2_DOT_DOT"
  [SM_BUS] -> Bus Selector21/1
  [SL_BUS] -> Bus Selector4/1
  [SL_BUS] -> Bus Selector22/1
  [SM_BUS] -> Bus Selector23/1
  [SL_BUS] -> Bus Selector24/1
  Bus Selector4/1 -> Mux12/1  "<TH4>"
  Bus Selector21/1 -> Mux12/2  "<TH4>"
  Bus Selector22/1 -> Mux13/1  "<TH4_D>"
  Bus Selector23/1 -> Mux13/2  "<TH4_D>"
  Bus Selector24/1 -> Mux11/1  "<TH4_DD>"
  Mux12/1 -> Bus Creator/10  "TH4"
  Mux13/1 -> Bus Creator/11  "TH4_DOT"
  Mux11/1 -> Bus Creator/12  "TH4_DOT_DOT"
  [SM_BUS] -> Bus Selector3/1
  Bus Selector3/1 -> Mux11/2  "<TH4_DD>"

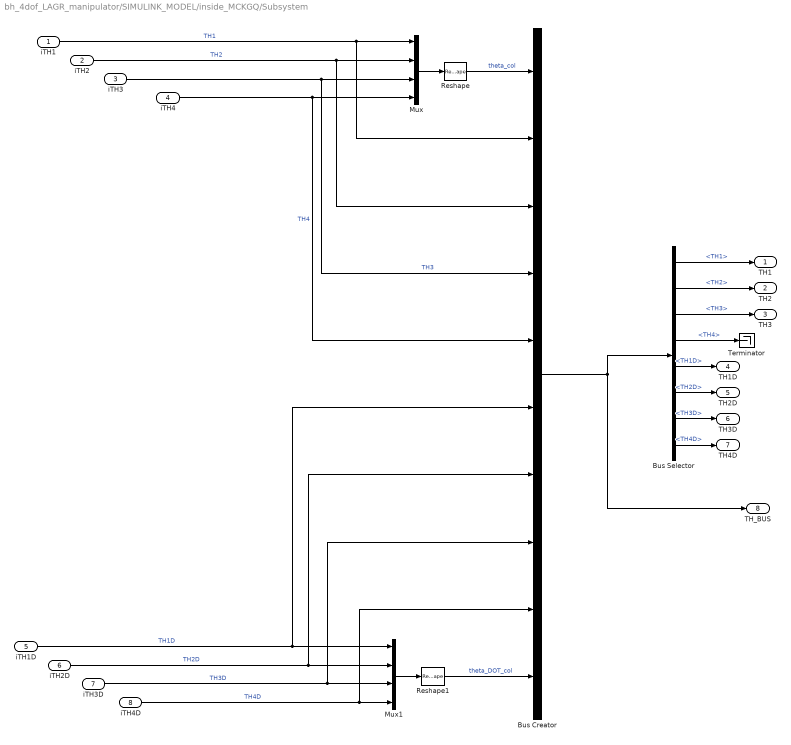
== system bh_4dof_LAGR_manipulator/SIMULINK_MODEL/inside_MCKGQ/Subsystem ==
  iTH1 : Inport
  iTH2 : Inport  Port=2
  iTH3 : Inport  Port=3
  iTH4 : Inport  Port=4
  iTH1D : Inport  Port=5
  iTH2D : Inport  Port=6
  iTH3D : Inport  Port=7
  iTH4D : Inport  Port=8
  Bus Creator : BusCreator  Inputs=10
  Bus Selector : BusSelector  OutputSignals=TH1,TH2,TH3,TH4,TH1D,TH2D,TH3D,TH4D
  Mux : Mux
  Mux1 : Mux
  Reshape : Reshape  OutputDimensionality=Column vector (2-D)
  Reshape1 : Reshape  OutputDimensionality=Column vector (2-D)
  Terminator : Terminator
  TH1 : Outport
  TH2 : Outport  Port=2
  TH3 : Outport  Port=3
  TH1D : Outport  Port=4
  TH2D : Outport  Port=5
  TH3D : Outport  Port=6
  TH4D : Outport  Port=7
  TH_BUS : Outport  Port=8
  wires:
  iTH2/1 -> Bus Creator/3, Mux/2  "TH2"
  iTH1/1 -> Bus Creator/2, Mux/1  "TH1"
  iTH2D/1 -> Bus Creator/7, Mux1/2  "TH2D"
  iTH1D/1 -> Bus Creator/6, Mux1/1  "TH1D"
  Mux/1 -> Reshape/1
  Mux1/1 -> Reshape1/1
  Reshape/1 -> Bus Creator/1  "theta_col"
  Reshape1/1 -> Bus Creator/10  "theta_DOT_col"
  Bus Creator/1 -> TH_BUS/1, Bus Selector/1
  iTH3D/1 -> Bus Creator/8, Mux1/3  "TH3D"
  iTH3/1 -> Bus Creator/4, Mux/3  "TH3"
  Bus Selector/1 -> TH1/1  "<TH1>"
  Bus Selector/2 -> TH2/1  "<TH2>"
  Bus Selector/3 -> TH3/1  "<TH3>"
  Bus Selector/5 -> TH1D/1  "<TH1D>"
  Bus Selector/6 -> TH2D/1  "<TH2D>"
  Bus Selector/7 -> TH3D/1  "<TH3D>"
  iTH4/1 -> Bus Creator/5, Mux/4  "TH4"
  iTH4D/1 -> Bus Creator/9, Mux1/4  "TH4D"
  Bus Selector/4 -> Terminator/1  "<TH4>"
  Bus Selector/8 -> TH4D/1  "<TH4D>"

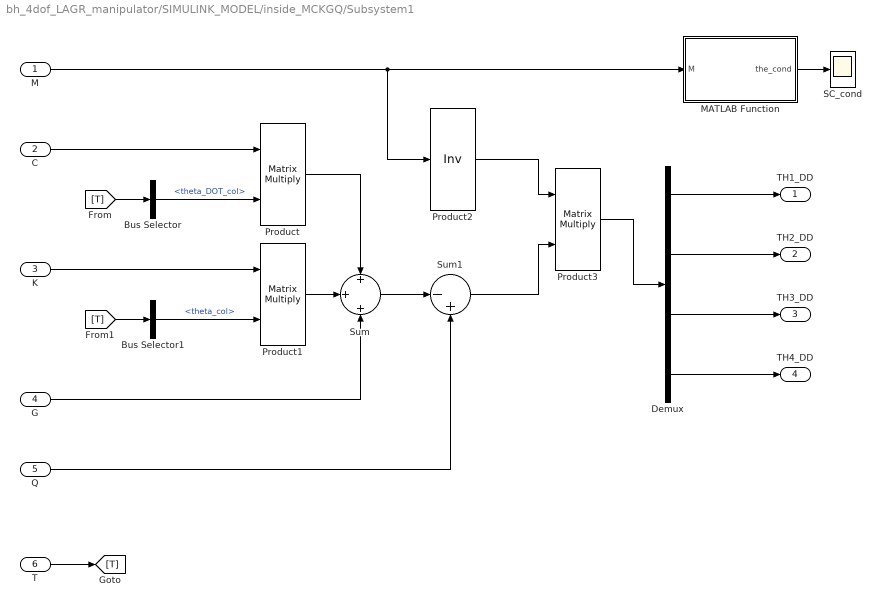
== system bh_4dof_LAGR_manipulator/SIMULINK_MODEL/inside_MCKGQ/Subsystem1 ==
  M : Inport
  C : Inport  Port=2
  K : Inport  Port=3
  G : Inport  Port=4
  Q : Inport  Port=5
  T : Inport  Port=6
  Bus Selector : BusSelector  OutputSignals=theta_DOT_col
  Bus Selector1 : BusSelector  OutputSignals=theta_col
  Demux : Demux
  MATLAB Function : MATLAB Function  TreatAsAtomicUnit=on
  Product : Product  Multiplication=Matrix(*)
  Product1 : Product  Multiplication=Matrix(*)
  Product2 : Product  Inputs=/  Multiplication=Matrix(*)
  Product3 : Product  Multiplication=Matrix(*)
  SC_cond : Scope
  Sum : Sum  Inputs=+|+|+
  Sum1 : Sum  Inputs=|-+
  TH1_DD : Outport
  TH2_DD : Outport  Port=2
  TH3_DD : Outport  Port=3
  TH4_DD : Outport  Port=4
  wires:
  T/1 -> [T]
  C/1 -> Product/1
  [T] -> Bus Selector/1
  Bus Selector/1 -> Product/2  "<theta_DOT_col>"
  K/1 -> Product1/1
  [T] -> Bus Selector1/1
  Bus Selector1/1 -> Product1/2  "<theta_col>"
  Q/1 -> Sum1/2
  Product1/1 -> Sum/2
  G/1 -> Sum/3
  Product/1 -> Sum/1
  Sum/1 -> Sum1/1
  M/1 -> Product2/1, MATLAB Function/1(M)
  Product2/1 -> Product3/1
  Sum1/1 -> Product3/2
  Product3/1 -> Demux/1
  Demux/1 -> TH1_DD/1
  Demux/2 -> TH2_DD/1
  MATLAB Function/1(the_cond) -> SC_cond/1
  Demux/3 -> TH3_DD/1
  Demux/4 -> TH4_DD/1
